simulink model "AlignTestMdl"  (R2012b)
settings: Solver=ode45  StartTime=0.0  StopTime=10.0  RelTol=1e-3
settings Model: Creator=henok.fessehatsion  LastModifiedBy=henok.fessehatsion

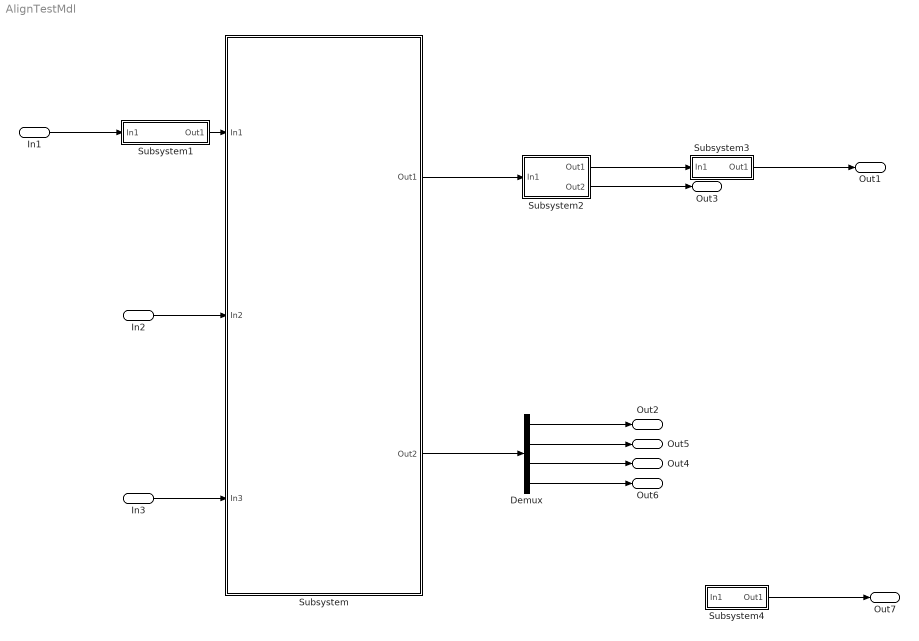
== system AlignTestMdl ==
  In1 : Inport
  In2 : Inport  Port=2
  In3 : Inport  Port=3
  Demux : Demux
  Subsystem : Subsystem
  Subsystem1 : Subsystem
  Subsystem2 : Subsystem
  Subsystem3 : Subsystem
  Subsystem4 : Subsystem
  Out1 : Outport
  Out2 : Outport  Port=2
  Out3 : Outport  Port=3
  Out4 : Outport  Port=4
  Out5 : Outport  Port=5
  Out6 : Outport  Port=6
  Out7 : Outport  Port=7
  wires:
  In1/1 -> Subsystem1/1(In1)
  In2/1 -> Subsystem/2(In2)
  In3/1 -> Subsystem/3(In3)
  Subsystem/1(Out1) -> Subsystem2/1(In1)
  Subsystem1/1(Out1) -> Subsystem/1(In1)
  Subsystem2/1(Out1) -> Subsystem3/1(In1)
  Subsystem3/1(Out1) -> Out1/1
  Subsystem2/2(Out2) -> Out3/1
  Subsystem/2(Out2) -> Demux/1
  Demux/4 -> Out6/1
  Demux/3 -> Out4/1
  Demux/2 -> Out5/1
  Demux/1 -> Out2/1
  Subsystem4/1(Out1) -> Out7/1

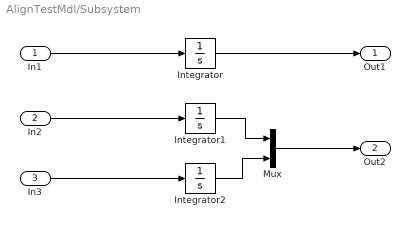
== system AlignTestMdl/Subsystem ==
  In1 : Inport
  In2 : Inport  Port=2
  In3 : Inport  Port=3
  Integrator : Integrator
  Integrator1 : Integrator
  Integrator2 : Integrator
  Mux : Mux  Inputs=2
  Out1 : Outport
  Out2 : Outport  Port=2
  wires:
  In3/1 -> Integrator2/1
  In1/1 -> Integrator/1
  In2/1 -> Integrator1/1
  Integrator/1 -> Out1/1
  Integrator1/1 -> Mux/1
  Mux/1 -> Out2/1
  Integrator2/1 -> Mux/2

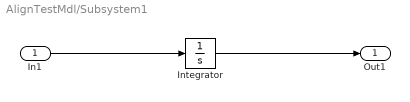
== system AlignTestMdl/Subsystem1 ==
  In1 : Inport
  Integrator : Integrator
  Out1 : Outport
  wires:
  Integrator/1 -> Out1/1
  In1/1 -> Integrator/1

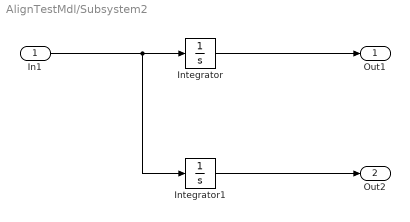
== system AlignTestMdl/Subsystem2 ==
  In1 : Inport
  Integrator : Integrator
  Integrator1 : Integrator
  Out1 : Outport
  Out2 : Outport  Port=2
  wires:
  Integrator/1 -> Out1/1
  In1/1 -> Integrator1/1, Integrator/1
  Integrator1/1 -> Out2/1

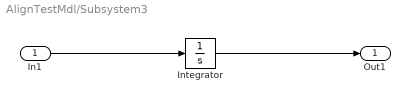
== system AlignTestMdl/Subsystem3 ==
  In1 : Inport
  Integrator : Integrator
  Out1 : Outport
  wires:
  In1/1 -> Integrator/1
  Integrator/1 -> Out1/1

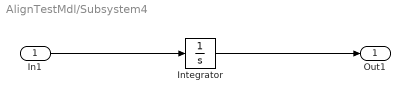
== system AlignTestMdl/Subsystem4 ==
  In1 : Inport
  Integrator : Integrator
  Out1 : Outport
  wires:
  Integrator/1 -> Out1/1
  In1/1 -> Integrator/1
